simulink model "Simulink_Matlab_Test"  (R2018b)
settings: Solver=VariableStepAuto  StartTime=0.0  StopTime=10.0  RelTol=1e-3
libraries: simulink x1
settings Model: Creator=James  LastModifiedBy=James

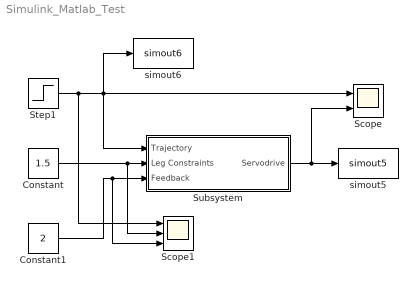
== system Simulink_Matlab_Test ==
  Constant : Constant  Value=1.5
  Constant1 : Constant  Value=2
  Scope : Scope  NumInputPorts=2
  Scope1 : Scope  NumInputPorts=3
  Step1 : Step  Time=2  SampleTime=0
  Subsystem : Subsystem
  simout5 : ToWorkspace  VariableName=simout5  SaveFormat=Timeseries  SampleTime=-1
  simout6 : ToWorkspace  VariableName=simout6  SaveFormat=Timeseries  SampleTime=-1
  wires:
  Constant1/1 -> Scope1/3, Subsystem/3(Feedback)
  Constant/1 -> Subsystem/2(Leg Constraints), Scope1/2
  Step1/1 -> Scope/1, simout6/1, Subsystem/1(Trajectory), Scope1/1
  Subsystem/1(Servodrive) -> simout5/1, Scope/2

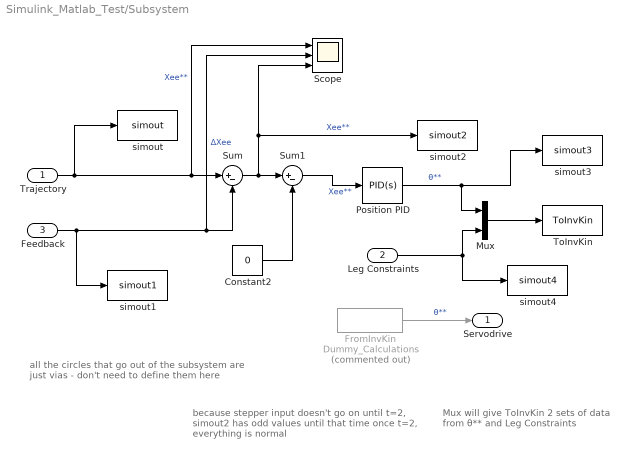
== system Simulink_Matlab_Test/Subsystem ==
  note: because stepper input doesn't go on until t=2,
      | simout2 has odd values until that time
      | once t=2, everything is normal
  note: Mux will give ToInvKin 2 sets of data
      | from θ** and Leg Constraints
  note: all the circles that go out of the subsystem
      | are just vias - don't need to define them here
  Trajectory : Inport
  Leg Constraints : Inport  Port=2
  Feedback : Inport  Port=3
  Constant2 : Constant  Value=0
  FromInvKin : FromWorkspace  Commented=on  VariableName=Dummy_Calculations  SampleTime=0
  Mux : Mux  Inputs=2
  Position PID : simulink/Continuous/PID Controller  Controller=PID  Form=Parallel  TimeDomain=Continuous-time  SampleTime=-1  IntegratorMethod=Forward Euler  FilterMethod=Forward Euler  ControllerParametersSource=internal  P=1  I=1  D=0  UseFilter=on  N=100  TunerSelectOption=Transfer Function Based (PID Tuner App)  InitialConditionSource=internal  InitialConditionForIntegrator=0  InitialConditionForFilter=0  DifferentiatorICPrevScaledInput=0  ExternalReset=none  TrackingMode=off  Kt=1  LimitOutput=off  UpperSaturationLimit=inf  LowerSaturationLimit=-inf  LinearizeAsGain=on  AntiWindupMode=none  Kb=1  POutMin=[]  POutMax=[]  IOutMin=[]  IOutMax=[]  DOutMin=[]  DOutMax=[]  NOutMin=[]  NOutMax=[]  SumOutMin=[]  SumOutMax=[]  SaturationOutMin=[]  SaturationOutMax=[]  PParamMin=[]  PParamMax=[]  IParamMin=[]  IParamMax=[]  DParamMin=[]  DParamMax=[]  NParamMin=[]  NParamMax=[]  KbParamMin=[]  KbParamMax=[]  KtParamMin=[]  KtParamMax=[]  KbOutMin=[]  KbOutMax=[]  KtOutMin=[]  KtOutMax=[]  IntegratorOutMin=[]  IntegratorOutMax=[]  FilterOutMin=[]  FilterOutMax=[]  SumI1OutMin=[]  SumI1OutMax=[]  SumI2OutMin=[]  SumI2OutMax=[]  SumI3OutMin=[]  SumI3OutMax=[]  SumI4OutMin=[]  SumI4OutMax=[]  SumDOutMin=[]  SumDOutMax=[]  DifferentiatorOutMin=[]  DifferentiatorOutMax=[]  FilterDiffOutCoefMin=[]  FilterDiffOutCoefMax=[]  ReciprocalOutMin=[]  ReciprocalOutMax=[]  SumDenOutMin=[]  SumDenOutMax=[]  SumNumOutMin=[]  SumNumOutMax=[]  DivideOutMin=[]  DivideOutMax=[]  IntegratorContinuousStateAttributes=''  IntegratorStateMustResolveToSignalObject=off  IntegratorRTWStateStorageClass=Auto  FilterContinuousStateAttributes=''  FilterStateMustResolveToSignalObject=off  FilterRTWStateStorageClass=Auto  ParallelPVariant=InternalParameters  IdealPVariant=Disabled  IVariant=InternalParameters  DVariant=InternalParameters  IntegratorVariant=Continuous  SatVariant=Disabled  AWVariant=Passthrough  PCopyVariant=Disabled  TRVariant=Disabled  FdbkBlocksVariant=Forward  IdealPFdbkVariant=Disabled  SatFdbkVariant=Disabled  DerivativeFilterVariant=ContFilter  NVariant=InternalParameters  NCopyVariant=Disabled  FilterICVariant=InternalICsFilter  IntegratorICVariant=InternalICs  ExternalResetVariant=Disabled  TRSumVariant=Passthrough  SumFdbkVariant=Disabled  SumVariant=Sum_PID
  Scope : Scope  NumInputPorts=3
  Sum : Sum  Inputs=|+-  InputSameDT=on
  Sum1 : Sum  Inputs=|+-  InputSameDT=on
  ToInvKin : ToWorkspace  VariableName=ToInvKin  SaveFormat=Timeseries  SampleTime=-1
  simout : ToWorkspace  VariableName=simout  SaveFormat=Timeseries  SampleTime=-1
  simout1 : ToWorkspace  VariableName=simout1  SaveFormat=Timeseries  SampleTime=-1
  simout2 : ToWorkspace  VariableName=simout2  SaveFormat=Timeseries  SampleTime=-1
  simout3 : ToWorkspace  VariableName=simout3  SaveFormat=Timeseries  SampleTime=-1
  simout4 : ToWorkspace  VariableName=simout4  SaveFormat=Timeseries  SampleTime=-1
  Servodrive : Outport
  wires:
  Position PID/1 -> simout3/1, Mux/1  "θ**"
  Mux/1 -> ToInvKin/1
  FromInvKin/1 -> Servodrive/1  "θ**"
  Leg Constraints/1 -> simout4/1, Mux/2
  Feedback/1 -> Sum/2, Scope/2, simout1/1  "ΔXee"
  Trajectory/1 -> Sum/1, Scope/1, simout/1  "Xee**"
  Sum/1 -> Sum1/1, simout2/1, Scope/3  "Xee**"
  Sum1/1 -> Position PID/1  "Xee**"
  Constant2/1 -> Sum1/2
